simulink model "HalfBandDecimator_Ex1"  (R2023a)
settings: Solver=VariableStepAuto  StartTime=0.0  StopTime=0.5  RelTol=1e-3
undefined symbols (not defined in the file): firhalfband, None, S, vsva2197, xcvc1902
libraries: dspsrcs4 x2, aieDSP x1, dspmlti4 x1, vmcUtilities x1
settings Model: Creator=sdegala  LastModifiedBy=robg
settings ModelReferenceCC: EnableRefExpFcnMdlSchedulingChecks=on

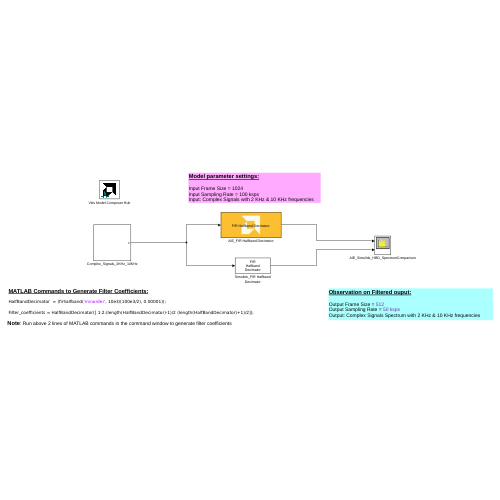
[thumbnail: Simulink's stored preview of the top-level diagram]
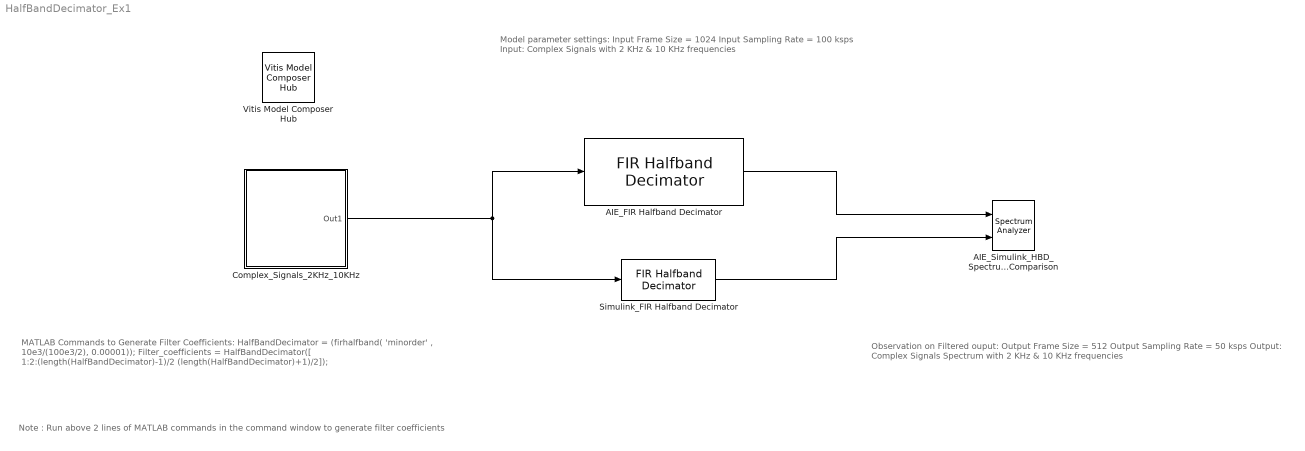
== system HalfBandDecimator_Ex1 ==
  note: MATLAB Commands to Generate Filter Coefficients:
      |
      | HalfBandDecimator = (firhalfband( 'minorder' , 10e3/(100e3/2), 0.00001));
      |
      | Filter_coefficients = HalfBandDecimator([ 1:2:(length(HalfBandDecimator)-1)/2 (length(HalfBandDecimator)+1)/2]);
  note: Note : Run above 2 lines of MATLAB commands in the command window to generate filter coefficients
  note: Model parameter settings:
      |
      | Input Frame Size = 1024
      | Input Sampling Rate = 100 ksps
      | Input: Complex Signals with 2 KHz & 10 KHz frequencies
  note: Observation on Filtered ouput:
      |
      | Output Frame Size = 512
      | Output Sampling Rate = 50 ksps
      | Output: Complex Signals Spectrum with 2 KHz & 10 KHz frequencies
  AIE_FIR Halfband Decimator : aieDSP/FIR Halfband Decimator  data_type=cfloat  coef_type=float  use_coeff_reload=off  dual_ip=off  num_outputs=off  coeff=Filter_coefficients  fir_length=31  input_window_size=1024  shift_val=0  rnd_mode=Round to positive infinity  sat_mode=0-None  deci_poly=1  casc_length=1  AIE_VARIANT=1  blockJsonConstraints=[]  blockJsonConstraintsInternal=[]  spec=vmc_fir_decimate_hb.json  SerializedMaskParamNames=[]  SerializedMaskParamValues=[]  SerializedMaskParamVisibilities=[]  block_type=FIR Halfband Decimator  SerializedMaskParamDataypes=typename|typename|bool|bool|bool|coef_type|uint|uint|uint|uint|uint|uint|uint|uint  SerializedMaskParamEnumStrArr=0|0|0|0|0|0|0|0|0|Floor,Ceiling,Round to positive infinity,Round to negative infinity,Round symmetrical to infinity,Round symmetrical to zero,Round convergent to even,Round convergent to odd|0-None,1-Asymmetric,3-Symmetric|0|0|0  SerializedMaskParamEnumValArr=0|0|0|0|0|0|0|0|0|0,1,2,3,4,5,6,7|0,1,3|0|0|0  SerializedMaskParamVectorArr=0|0|0|0|0|1|0|0|0|0|0|0|0|0
  AIE_Simulink_HBD_SpectrumComparison : SpectrumAnalyzer  NumInputPorts=2  AveragingMethod=Exponential  ShowLegend=on  ChannelNames="[\"\"]"  DefaultConfigurationName=spbscopes.SpectrumAnalyzerBlockCfg
  Complex_Signals_2KHz_10KHz : Subsystem
  Simulink_FIR Halfband Decimator : dspmlti4/FIR Halfband Decimator  InheritSampleRate=on  Specification=Coefficients  FilterOrder=52  TransitionWidth=4.1e3  StopbandAttenuation=80  DesignMethod=Auto  Numerator=firhalfband('minorder', 10e3/(100e3/2), 0.00001)  FilterBankOutputPort=off  SampleRate=125e3  SimulateUsing=Code generation  roundingMode=Ceiling  coeffsDataTypeStr=fixdt(1,32)
  Vitis Model Composer Hub : vmcUtilities/Vitis Model Composer Hub  Tag=genX  CodeGeneration=off  StartColumn=1  NumberOfColumns=1  TargetDirectory=./code  exportDesign=off  analyzeDesign=off  validateDesignOnHw=off  ExportType=AI Engines  IpVendor=xilinx.com  IpLibrary=hls  IpVersion=1.0  IpHWLanguage=Verilog  AieCompilerOptions={}  AieSimulatorOptions={}  CreateTestbench=off  TestbenchStackSize=10  RunRtlSim=off  RunCSim=off  RunAieSim=off  AieSimTimeout=50000  RunAieSimProfiling=off  LaunchVitisAnalyzer=off  PlotOutput=off  RunX86Sim=off  X86SimTimeout=10  GenHwImage=off  GenLibadfXo=off  GenHwValidationCode=off  PlatformType=Not Specified  HwSystemType=Baremetal  HwValidationTarget=hw  ProjDevice=xcvc1902-vsva2197-1LP-e-S  ProjDevicePart=xcvc1902-vsva2197-1LP-e-S  AIEType=AIE  SamplePeriod=-1  ClockFrequency=200  DataPathParallelism=1  xilinxfamily=versalaicore  part=xcvc1902  speed=-1LP-e-S  package=vsva2197  directory=./netlist  testbench=off  incr_netlist=off  synthesis_tool=Vivado  clock_wrapper=Clock Enables  dbl_ovrd=According to Block Masks  dcm_input_clock_period=10  sysclk_period=10  simulink_period=1  eval_field=0  LogFileName=''  NThreads=4
  wires:
  Simulink_FIR Halfband Decimator/1 -> AIE_Simulink_HBD_SpectrumComparison/2
  Complex_Signals_2KHz_10KHz/1(Out1) -> Simulink_FIR Halfband Decimator/1, AIE_FIR Halfband Decimator/1
  AIE_FIR Halfband Decimator/1 -> AIE_Simulink_HBD_SpectrumComparison/1

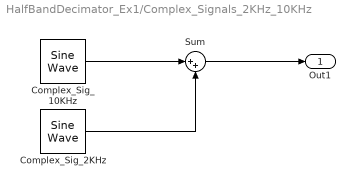
== system HalfBandDecimator_Ex1/Complex_Signals_2KHz_10KHz ==
  Complex_Sig_10KHz : dspsrcs4/Sine Wave  Amplitude=0.5  Frequency=10e3  Phase=0  SampleMode=Discrete  OutComplex=Complex  CompMethod=Trigonometric fcn  TableSize=Speed  SampleTime=1/100e3  SamplesPerFrame=1024  ResetState=Restart at time zero  OutputFrames=off  dataType=single  wordLen=16  udDataType=sfix(16)  fracBitsMode=Best precision  numFracBits=15  OutDataTypeStr=single  LastOutDataTypeStr=single
  Complex_Sig_2KHz : dspsrcs4/Sine Wave  Amplitude=1  Frequency=2e3  Phase=0  SampleMode=Discrete  OutComplex=Complex  CompMethod=Trigonometric fcn  TableSize=Speed  SampleTime=1/100e3  SamplesPerFrame=1024  ResetState=Restart at time zero  OutputFrames=off  dataType=single  wordLen=16  udDataType=sfix(16)  fracBitsMode=Best precision  numFracBits=15  OutDataTypeStr=single  LastOutDataTypeStr=single
  Sum : Sum  Inputs=|++
  Out1 : Outport
  wires:
  Complex_Sig_2KHz/1 -> Sum/2
  Complex_Sig_10KHz/1 -> Sum/1
  Sum/1 -> Out1/1
